simulink model "multiple_generators_els_2018b"  (Simulink 9.2)
settings: Solver=ode15s  StartTime=0.0  StopTime=4000  RelTol=1e-3
InitFcn:
  | global LOData LOModelData gprMdlLP_machine1 gprMdlLP_machine2 gprMdlLP_machine3 gprMdlLP_machine4 gprMdlLP_machine5 significance SteadyState explore explore_signal total_uncertainty
  | load load_opt_multiple_init2.mat
undefined symbols (not defined in the file or in its folder): sigbuilder_block
libraries: simulink x10
settings Model: Creator=Memo Mer  LastModifiedBy=mmercang
settings DataIOCC: LimitDataPoints=off  SaveFormat=Dataset  SignalLoggingSaveFormat=Dataset  ReturnWorkspaceOutputs=on
settings OptimizationCC: LifeSpan=auto
settings DebuggingCC: UnderspecifiedInitializationDetection=Simplified  MergeDetectMultiDrivingBlocksExec=error  FcnCallInpInsideContextMsg=error  StateNameClashWarn=none  SFUnexpectedBacktrackingDiag=error  SFNoUnconditionalDefaultTransitionDiag=error  SFExecutionAtInitializationDiag=warning
settings HardwareCC: ProdBitPerPointer=64  ProdBitPerSizeT=64  ProdBitPerPtrDiffT=64  ProdLargestAtomicFloat=Float  ProdIntDivRoundTo=Zero  ProdEndianess=LittleEndian  ProdWordSize=64  ProdHWDeviceType=Intel->x86-64 (Windows64)
settings ModelReferenceCC: PropagateSignalLabelsOutOfModel=on
settings SFSimCC: SimUseLocalCustomCode=on
settings RTWCC: RTWUseLocalCustomCode=on
settings CodeAppCC: StateflowObjectComments=off
settings GRTTargetCC: TargetLangStandard=C99 (ISO)  CombineOutputUpdateFcns=on  GRTInterface=off
settings ConfigComp: CovMetricSettings=dwe  CovSaveCumulativeToWorkspaceVar=off  CovSaveSingleToWorkspaceVar=off  CovExternalEMLEnable=on

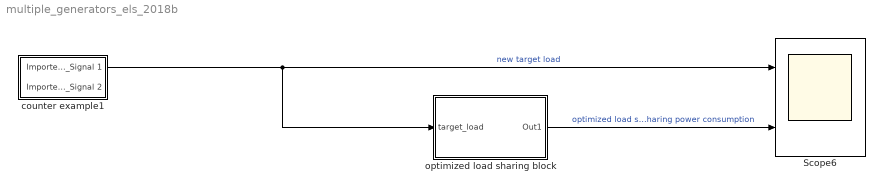
== system multiple_generators_els_2018b ==
  Scope6 : Scope  NumInputPorts=2
  counter example1 : Subsystem  Tag=STV Subsys  LoadFcn=sigbuilder_block('load');  StartFcn=sigbuilder_block('start');  StopFcn=sigbuilder_block('stop');  ClipboardFcn=sigbuilder_block('clipboard');  mask(Sigbuilder block){tuvar=[0:10]}
      mask help: Simulink:masks:SigbuilderBlock_MD
      mask init:
      | if ~strcmp(get_param(bdroot(gcbh),'SimulationStatus'),'stopped') tuvar = sigbuilder_block('maskInit'); end
      settings: CopyFcn=sigbuilder_block('copy');  DeleteFcn=sigbuilder_block('delete');  ModelCloseFcn=sigbuilder_block('modelClose');  PreSaveFcn=sigbuilder_block('preSave');  PauseFcn=sigbuilder_block('pause');  ContinueFcn=sigbuilder_block('continue');  NameChangeFcn=sigbuilder_block('namechange');  OpenFcn=sigbuilder_block('open',[384 46.5 890 699.75 ]);  CloseFcn=sigbuilder_block('close');
      mask Display: plot(0, 0, 100, 100,[2, 2, 32, 32, 2], [68, 8, 8, 68, 68],[32, 2], [38, 38], [32, 19, 2],[53, 60, 44], [32, 17, 17, 2],[16, 16, 31, 31]);txt = getActiveGroup(gcbh);text(2, 100, txt,'verticalAlignment', 'top');
  optimized load sharing block : Subsystem  Tag=equal load sharing
  wires:
  counter example1/1(Imported_Signal 1) -> optimized load sharing block/1(target_load), Scope6/1  "new target load"
  optimized load sharing block/1(Out1) -> Scope6/2  "optimized load sharing power consumption"

== system multiple_generators_els_2018b/counter example1 ==
  Demux : Demux  Tag=STV Demux  Outputs=2
      settings: DisplayOption=none
  FromWs : FromWorkspace  Tag=STV FromWs  VariableName=tuvar  SigBuilderData=DataTag0  VnvData=DataTag1
      SigBuilderData=|
      | common.afterFinalStr = 'Extrapolate'
      | common.sampleTime = '0'
      | dataSet.timeRange = [0 7000]
      | dataSet.name = 'Imported_Group 1'
      | sbobj.Groups.Name = 'Imported_Group 1'
      | sbobj.Groups.Signals(1).Name = 'Imported_Signal 1'
      | sbobj.Groups.Signals(1).XData = [0 1000 1000 2000 2000 3000 4000 4000 5000 5000 6000 6000 7000]
      | sbobj.Groups.Signals(1).YData = [830 830 1035 1035 2500 2500 2500 1830 1830 1170 1170 1660 1660]
      | sbobj.Groups.Signals(2).Name = 'Imported_Signal 2'
      | sbobj.Groups.Signals(2).XData = [0 1000 2000 3000 4000 5000 6000 7000]
      | sbobj.Groups.Signals(2).YData = [1800 1800 1800 1800 1800 1800 1800 1800]
      | sbobj.Groups.TimeRange = [0 7000]
  Imported_Signal 1 : Outport  Tag=STV Outport
  Imported_Signal 2 : Outport  Tag=STV Outport  Port=2
  wires:
  Demux/2 -> Imported_Signal 2/1
  Demux/1 -> Imported_Signal 1/1
  FromWs/1 -> Demux/1

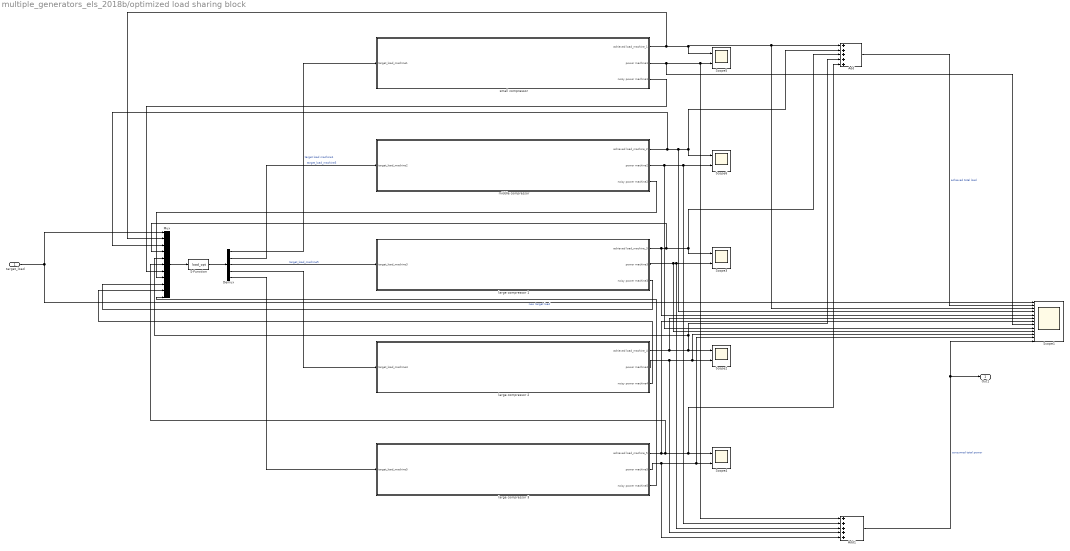
== system multiple_generators_els_2018b/optimized load sharing block ==
  target_load : Inport
  Add : Sum  Inputs=+++++
  Add1 : Sum  Inputs=+++++
  Demux : Demux  Outputs=5
  Mux : Mux  Inputs=11
  S-Function : S-Function  FunctionName=load_opt  Parameters=[],[]  SFunctionDeploymentMode=off  EnableBusSupport=off
  Scope1 : Scope  NumInputPorts=13
  Scope{2..6} (5 alike) : Scope  NumInputPorts=2
  large compressor 1 : Subsystem
  large compressor 2 : Subsystem
  large compressor 3 : Subsystem
  middle compressor : Subsystem
  small compressor : Subsystem
  Out1 : Outport
  wires:
  Add/1 -> Scope1/2  "achieved total load"
  Add1/1 -> Out1/1, Scope1/13  "consumed total power"
  Mux/1 -> S-Function/1
  target_load/1 -> Mux/1, Scope1/1  "new target load"
  S-Function/1 -> Demux/1
  large compressor 1/1(achieved load_machine_3) -> Scope1/5, Mux/4, Scope3/1, Add/3
  large compressor 3/1(achieved load_machine_5) -> Scope1/7, Mux/6, Add/5, Scope4/1
  large compressor 3/2(power machine5) -> Add1/5, Scope1/12, Scope4/2
  middle compressor/1(achieved load_machine_2) -> Scope1/4, Scope6/1, Add/2, Mux/3
  middle compressor/2(power machine2) -> Scope1/9, Add1/2, Scope6/2
  small compressor/2(power machine1) -> Scope1/8, Add1/1, Scope5/2
  Demux/1 -> small compressor/1(target_load_machine1)  "target load machine1"
  Demux/2 -> middle compressor/1(target_load_machine2)  "target_load_machine5"
  Demux/3 -> large compressor 1/1(target_load_machine3)  "target_load_machine5"
  Demux/4 -> large compressor 2/1(target_load_machine4)
  Demux/5 -> large compressor 3/1(target_load_machine5)
  large compressor 3/3(noisy power machine5) -> Mux/11
  large compressor 2/3(noisy power machine4) -> Mux/10
  middle compressor/3(noisy power machine2) -> Mux/8
  large compressor 1/3(noisy power machine3) -> Mux/9
  small compressor/3(noisy power machine1) -> Mux/7
  small compressor/1(achieved load_machine_1) -> Scope5/1, Scope1/3, Add/1, Mux/2
  large compressor 1/2(power machine3) -> Scope1/10, Add1/3, Scope3/2
  large compressor 2/1(achieved load_machine_4) -> Scope1/6, Add/4, Mux/5, Scope2/1
  large compressor 2/2(power machine4) -> Add1/4, Scope1/11, Scope2/2

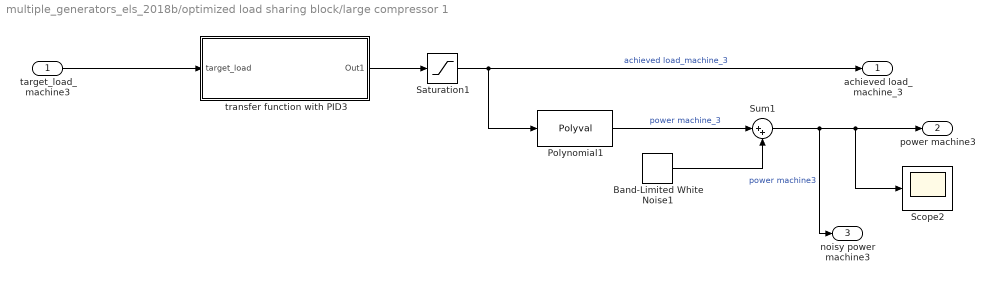
== system multiple_generators_els_2018b/optimized load sharing block/large compressor 1 ==
  target_load_machine3 : Inport
  Band-Limited White Noise1 : simulink/Sources/Band-Limited White Noise  Cov=[0.1]  Ts=5  seed=[23341]
  Polynomial1 : Polyval  Coefs="[-1.53490519e-09  2.28838030e-06 -9.59520873e-04 6.18821903e-01 7.51758182e+01]"
  Saturation1 : Saturate  UpperLimit=795  LowerLimit=194
  Scope2 : Scope
  Sum1 : Sum  Inputs=|++
  transfer function with PID3 : Subsystem
  achieved load_machine_3 : Outport
  power machine3 : Outport  Port=2
  noisy power machine3 : Outport  Port=3
  wires:
  Polynomial1/1 -> Sum1/1  "power machine_3"
  target_load_machine3/1 -> transfer function with PID3/1(target_load)
  transfer function with PID3/1(Out1) -> Saturation1/1
  Band-Limited White Noise1/1 -> Sum1/2
  Saturation1/1 -> achieved load_machine_3/1, Polynomial1/1  "achieved load_machine_3"
  Sum1/1 -> noisy power machine3/1, power machine3/1, Scope2/1  "power machine3"

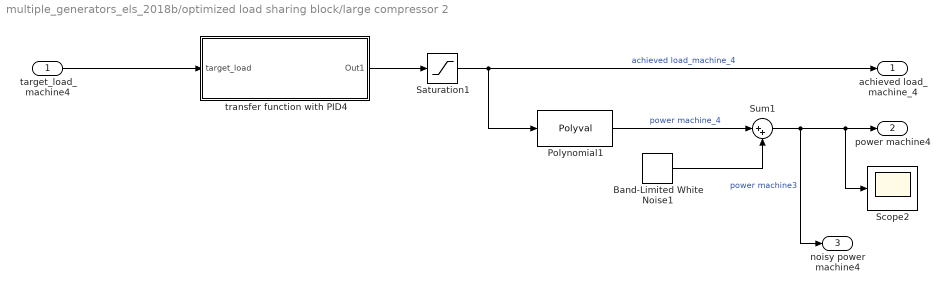
== system multiple_generators_els_2018b/optimized load sharing block/large compressor 2 ==
  target_load_machine4 : Inport
  Band-Limited White Noise1 : simulink/Sources/Band-Limited White Noise  Cov=[0.1]  Ts=5  seed=[23341]
  Polynomial1 : Polyval  Coefs="[-1.53490519e-09  2.28838030e-06 -9.59520873e-04 6.18821903e-01 7.51758182e+01]"
  Saturation1 : Saturate  UpperLimit=795  LowerLimit=194
  Scope2 : Scope
  Sum1 : Sum  Inputs=|++
  transfer function with PID4 : Subsystem
  achieved load_machine_4 : Outport
  power machine4 : Outport  Port=2
  noisy power machine4 : Outport  Port=3
  wires:
  Polynomial1/1 -> Sum1/1  "power machine_4"
  Sum1/1 -> power machine4/1, Scope2/1, noisy power machine4/1  "power machine3"
  target_load_machine4/1 -> transfer function with PID4/1(target_load)
  transfer function with PID4/1(Out1) -> Saturation1/1
  Band-Limited White Noise1/1 -> Sum1/2
  Saturation1/1 -> achieved load_machine_4/1, Polynomial1/1  "achieved load_machine_4"

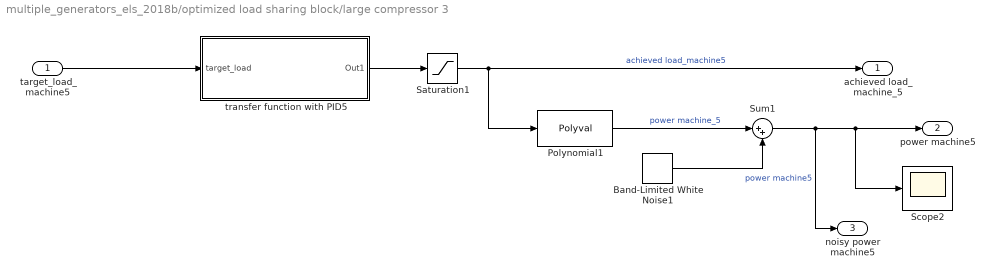
== system multiple_generators_els_2018b/optimized load sharing block/large compressor 3 ==
  target_load_machine5 : Inport
  Band-Limited White Noise1 : simulink/Sources/Band-Limited White Noise  Cov=[0.1]  Ts=5  seed=[23341]
  Polynomial1 : Polyval  Coefs="[-1.53490519e-09  2.28838030e-06 -9.59520873e-04 6.18821903e-01 7.51758182e+01]"
  Saturation1 : Saturate  UpperLimit=795  LowerLimit=194
  Scope2 : Scope
  Sum1 : Sum  Inputs=|++
  transfer function with PID5 : Subsystem
  achieved load_machine_5 : Outport
  power machine5 : Outport  Port=2
  noisy power machine5 : Outport  Port=3
  wires:
  Polynomial1/1 -> Sum1/1  "power machine_5"
  target_load_machine5/1 -> transfer function with PID5/1(target_load)
  transfer function with PID5/1(Out1) -> Saturation1/1
  Band-Limited White Noise1/1 -> Sum1/2
  Saturation1/1 -> achieved load_machine_5/1, Polynomial1/1  "achieved load_machine5"
  Sum1/1 -> power machine5/1, Scope2/1, noisy power machine5/1  "power machine5"

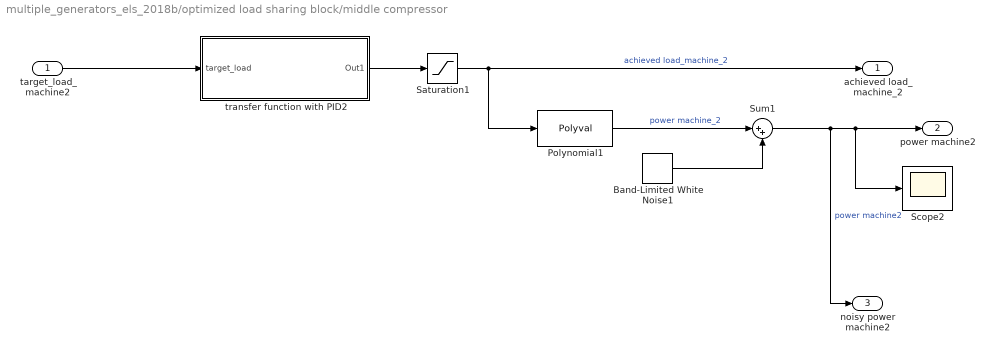
== system multiple_generators_els_2018b/optimized load sharing block/middle compressor ==
  target_load_machine2 : Inport
  Band-Limited White Noise1 : simulink/Sources/Band-Limited White Noise  Cov=[0.1]  Ts=5  seed=[23341]
  Polynomial1 : Polyval  Coefs=[-1.42718017e-08 1.87477980e-05 -8.28649653e-03 1.88469092 -2.19952823]
  Saturation1 : Saturate  UpperLimit=537  LowerLimit=237
  Scope2 : Scope
  Sum1 : Sum  Inputs=|++
  transfer function with PID2 : Subsystem
  achieved load_machine_2 : Outport
  power machine2 : Outport  Port=2
  noisy power machine2 : Outport  Port=3
  wires:
  Polynomial1/1 -> Sum1/1  "power machine_2"
  target_load_machine2/1 -> transfer function with PID2/1(target_load)
  transfer function with PID2/1(Out1) -> Saturation1/1
  Band-Limited White Noise1/1 -> Sum1/2
  Saturation1/1 -> achieved load_machine_2/1, Polynomial1/1  "achieved load_machine_2"
  Sum1/1 -> noisy power machine2/1, power machine2/1, Scope2/1  "power machine2"

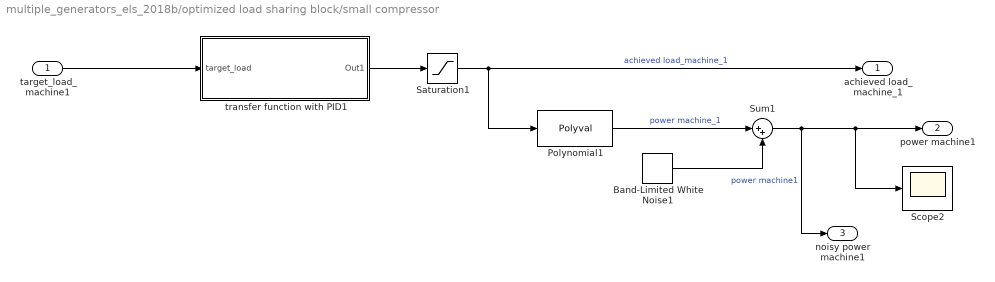
== system multiple_generators_els_2018b/optimized load sharing block/small compressor ==
  target_load_machine1 : Inport
  Band-Limited White Noise1 : simulink/Sources/Band-Limited White Noise  Cov=[0.1]  Ts=5  seed=[23341]
  Polynomial1 : Polyval  Coefs=[-9e-08 4e-05 -0.0052 0.7765 15.661]
  Saturation1 : Saturate  UpperLimit=220  LowerLimit=56
  Scope2 : Scope
  Sum1 : Sum  Inputs=|++
  transfer function with PID1 : Subsystem
  achieved load_machine_1 : Outport
  power machine1 : Outport  Port=2
  noisy power machine1 : Outport  Port=3
  wires:
  Polynomial1/1 -> Sum1/1  "power machine_1"
  target_load_machine1/1 -> transfer function with PID1/1(target_load)
  transfer function with PID1/1(Out1) -> Saturation1/1
  Band-Limited White Noise1/1 -> Sum1/2
  Saturation1/1 -> achieved load_machine_1/1, Polynomial1/1  "achieved load_machine_1"
  Sum1/1 -> power machine1/1, Scope2/1, noisy power machine1/1  "power machine1"

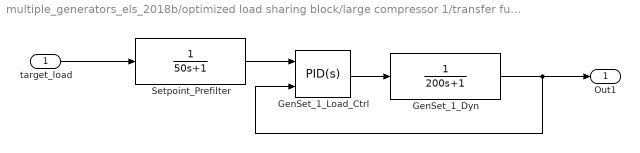
== system multiple_generators_els_2018b/optimized load sharing block/large compressor 1/transfer function with PID3 ==
  target_load : Inport
  GenSet_1_Dyn : TransferFcn  Denominator=[200 1]
  GenSet_1_Load_Ctrl : simulink/Continuous/PID Controller (2DOF)  Controller=PID  Form=Parallel  TimeDomain=Continuous-time  SampleTime=-1  IntegratorMethod=Forward Euler  FilterMethod=Forward Euler  ControllerParametersSource=internal  P=100  I=10  D=0  UseFilter=on  N=100  b=1  c=1  TunerSelectOption=Transfer Function Based (PID Tuner App)  InitialConditionSource=internal  InitialConditionForIntegrator=0  InitialConditionForFilter=0  DifferentiatorICPrevScaledInput=0  ExternalReset=none  TrackingMode=off  Kt=1  LimitOutput=off  UpperSaturationLimit=inf  LowerSaturationLimit=-inf  LinearizeAsGain=on  AntiWindupMode=none  Kb=1  POutMin=[]  POutMax=[]  IOutMin=[]  IOutMax=[]  DOutMin=[]  DOutMax=[]  NOutMin=[]  NOutMax=[]  bOutMin=[]  bOutMax=[]  cOutMin=[]  cOutMax=[]  SumOutMin=[]  SumOutMax=[]  SaturationOutMin=[]  SaturationOutMax=[]  PParamMin=[]  PParamMax=[]  IParamMin=[]  IParamMax=[]  DParamMin=[]  DParamMax=[]  NParamMin=[]  NParamMax=[]  bParamMin=[]  bParamMax=[]  cParamMin=[]  cParamMax=[]  KbParamMin=[]  KbParamMax=[]  KtParamMin=[]  KtParamMax=[]  KbOutMin=[]  KbOutMax=[]  KtOutMin=[]  KtOutMax=[]  IntegratorOutMin=[]  IntegratorOutMax=[]  FilterOutMin=[]  FilterOutMax=[]  SumI1OutMin=[]  SumI1OutMax=[]  SumI2OutMin=[]  SumI2OutMax=[]  SumI3OutMin=[]  SumI3OutMax=[]  SumI4OutMin=[]  SumI4OutMax=[]  SumDOutMin=[]  SumDOutMax=[]  Sum1OutMin=[]  Sum1OutMax=[]  Sum2OutMin=[]  Sum2OutMax=[]  Sum3OutMin=[]  Sum3OutMax=[]  DifferentiatorOutMin=[]  DifferentiatorOutMax=[]  FilterDiffOutCoefMin=[]  FilterDiffOutCoefMax=[]  ReciprocalOutMin=[]  ReciprocalOutMax=[]  SumDenOutMin=[]  SumDenOutMax=[]  SumNumOutMin=[]  SumNumOutMax=[]  DivideOutMin=[]  DivideOutMax=[]  IntegratorContinuousStateAttributes=''  IntegratorStateMustResolveToSignalObject=off  IntegratorRTWStateStorageClass=Auto  FilterContinuousStateAttributes=''  FilterStateMustResolveToSignalObject=off  FilterRTWStateStorageClass=Auto  ParallelPVariant=InternalParameters  IdealPVariant=Disabled  IVariant=InternalParameters  DVariant=InternalParameters  bVariant=InternalParameters  cVariant=InternalParameters  IntegratorVariant=Continuous  SatVariant=Disabled  AWVariant=Passthrough  PCopyVariant=Disabled  TRVariant=Disabled  FdbkBlocksVariant=Forward  IdealPFdbkVariant=Disabled  SatFdbkVariant=Disabled  DerivativeFilterVariant=ContFilter  NVariant=InternalParameters  NCopyVariant=Disabled  FilterICVariant=InternalICsFilter  IntegratorICVariant=InternalICs  ExternalResetVariant=Disabled  TRSumVariant=Passthrough  SumFdbkVariant=Disabled  SumVariant=Sum_PID
  Setpoint_Prefilter : TransferFcn  Denominator=[50 1]
  Out1 : Outport
  wires:
  GenSet_1_Load_Ctrl/1 -> GenSet_1_Dyn/1
  Setpoint_Prefilter/1 -> GenSet_1_Load_Ctrl/1
  target_load/1 -> Setpoint_Prefilter/1
  GenSet_1_Dyn/1 -> Out1/1, GenSet_1_Load_Ctrl/2

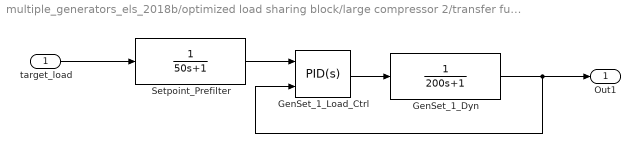
== system multiple_generators_els_2018b/optimized load sharing block/large compressor 2/transfer function with PID4 ==
  target_load : Inport
  GenSet_1_Dyn : TransferFcn  Denominator=[200 1]
  GenSet_1_Load_Ctrl : simulink/Continuous/PID Controller (2DOF)  Controller=PID  Form=Parallel  TimeDomain=Continuous-time  SampleTime=-1  IntegratorMethod=Forward Euler  FilterMethod=Forward Euler  ControllerParametersSource=internal  P=100  I=10  D=0  UseFilter=on  N=100  b=1  c=1  TunerSelectOption=Transfer Function Based (PID Tuner App)  InitialConditionSource=internal  InitialConditionForIntegrator=0  InitialConditionForFilter=0  DifferentiatorICPrevScaledInput=0  ExternalReset=none  TrackingMode=off  Kt=1  LimitOutput=off  UpperSaturationLimit=inf  LowerSaturationLimit=-inf  LinearizeAsGain=on  AntiWindupMode=none  Kb=1  POutMin=[]  POutMax=[]  IOutMin=[]  IOutMax=[]  DOutMin=[]  DOutMax=[]  NOutMin=[]  NOutMax=[]  bOutMin=[]  bOutMax=[]  cOutMin=[]  cOutMax=[]  SumOutMin=[]  SumOutMax=[]  SaturationOutMin=[]  SaturationOutMax=[]  PParamMin=[]  PParamMax=[]  IParamMin=[]  IParamMax=[]  DParamMin=[]  DParamMax=[]  NParamMin=[]  NParamMax=[]  bParamMin=[]  bParamMax=[]  cParamMin=[]  cParamMax=[]  KbParamMin=[]  KbParamMax=[]  KtParamMin=[]  KtParamMax=[]  KbOutMin=[]  KbOutMax=[]  KtOutMin=[]  KtOutMax=[]  IntegratorOutMin=[]  IntegratorOutMax=[]  FilterOutMin=[]  FilterOutMax=[]  SumI1OutMin=[]  SumI1OutMax=[]  SumI2OutMin=[]  SumI2OutMax=[]  SumI3OutMin=[]  SumI3OutMax=[]  SumI4OutMin=[]  SumI4OutMax=[]  SumDOutMin=[]  SumDOutMax=[]  Sum1OutMin=[]  Sum1OutMax=[]  Sum2OutMin=[]  Sum2OutMax=[]  Sum3OutMin=[]  Sum3OutMax=[]  DifferentiatorOutMin=[]  DifferentiatorOutMax=[]  FilterDiffOutCoefMin=[]  FilterDiffOutCoefMax=[]  ReciprocalOutMin=[]  ReciprocalOutMax=[]  SumDenOutMin=[]  SumDenOutMax=[]  SumNumOutMin=[]  SumNumOutMax=[]  DivideOutMin=[]  DivideOutMax=[]  IntegratorContinuousStateAttributes=''  IntegratorStateMustResolveToSignalObject=off  IntegratorRTWStateStorageClass=Auto  FilterContinuousStateAttributes=''  FilterStateMustResolveToSignalObject=off  FilterRTWStateStorageClass=Auto  ParallelPVariant=InternalParameters  IdealPVariant=Disabled  IVariant=InternalParameters  DVariant=InternalParameters  bVariant=InternalParameters  cVariant=InternalParameters  IntegratorVariant=Continuous  SatVariant=Disabled  AWVariant=Passthrough  PCopyVariant=Disabled  TRVariant=Disabled  FdbkBlocksVariant=Forward  IdealPFdbkVariant=Disabled  SatFdbkVariant=Disabled  DerivativeFilterVariant=ContFilter  NVariant=InternalParameters  NCopyVariant=Disabled  FilterICVariant=InternalICsFilter  IntegratorICVariant=InternalICs  ExternalResetVariant=Disabled  TRSumVariant=Passthrough  SumFdbkVariant=Disabled  SumVariant=Sum_PID
  Setpoint_Prefilter : TransferFcn  Denominator=[50 1]
  Out1 : Outport
  wires:
  GenSet_1_Load_Ctrl/1 -> GenSet_1_Dyn/1
  Setpoint_Prefilter/1 -> GenSet_1_Load_Ctrl/1
  target_load/1 -> Setpoint_Prefilter/1
  GenSet_1_Dyn/1 -> Out1/1, GenSet_1_Load_Ctrl/2

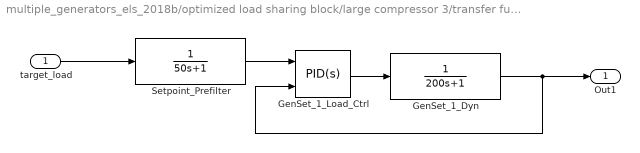
== system multiple_generators_els_2018b/optimized load sharing block/large compressor 3/transfer function with PID5 ==
  target_load : Inport
  GenSet_1_Dyn : TransferFcn  Denominator=[200 1]
  GenSet_1_Load_Ctrl : simulink/Continuous/PID Controller (2DOF)  Controller=PID  Form=Parallel  TimeDomain=Continuous-time  SampleTime=-1  IntegratorMethod=Forward Euler  FilterMethod=Forward Euler  ControllerParametersSource=internal  P=100  I=10  D=0  UseFilter=on  N=100  b=1  c=1  TunerSelectOption=Transfer Function Based (PID Tuner App)  InitialConditionSource=internal  InitialConditionForIntegrator=0  InitialConditionForFilter=0  DifferentiatorICPrevScaledInput=0  ExternalReset=none  TrackingMode=off  Kt=1  LimitOutput=off  UpperSaturationLimit=inf  LowerSaturationLimit=-inf  LinearizeAsGain=on  AntiWindupMode=none  Kb=1  POutMin=[]  POutMax=[]  IOutMin=[]  IOutMax=[]  DOutMin=[]  DOutMax=[]  NOutMin=[]  NOutMax=[]  bOutMin=[]  bOutMax=[]  cOutMin=[]  cOutMax=[]  SumOutMin=[]  SumOutMax=[]  SaturationOutMin=[]  SaturationOutMax=[]  PParamMin=[]  PParamMax=[]  IParamMin=[]  IParamMax=[]  DParamMin=[]  DParamMax=[]  NParamMin=[]  NParamMax=[]  bParamMin=[]  bParamMax=[]  cParamMin=[]  cParamMax=[]  KbParamMin=[]  KbParamMax=[]  KtParamMin=[]  KtParamMax=[]  KbOutMin=[]  KbOutMax=[]  KtOutMin=[]  KtOutMax=[]  IntegratorOutMin=[]  IntegratorOutMax=[]  FilterOutMin=[]  FilterOutMax=[]  SumI1OutMin=[]  SumI1OutMax=[]  SumI2OutMin=[]  SumI2OutMax=[]  SumI3OutMin=[]  SumI3OutMax=[]  SumI4OutMin=[]  SumI4OutMax=[]  SumDOutMin=[]  SumDOutMax=[]  Sum1OutMin=[]  Sum1OutMax=[]  Sum2OutMin=[]  Sum2OutMax=[]  Sum3OutMin=[]  Sum3OutMax=[]  DifferentiatorOutMin=[]  DifferentiatorOutMax=[]  FilterDiffOutCoefMin=[]  FilterDiffOutCoefMax=[]  ReciprocalOutMin=[]  ReciprocalOutMax=[]  SumDenOutMin=[]  SumDenOutMax=[]  SumNumOutMin=[]  SumNumOutMax=[]  DivideOutMin=[]  DivideOutMax=[]  IntegratorContinuousStateAttributes=''  IntegratorStateMustResolveToSignalObject=off  IntegratorRTWStateStorageClass=Auto  FilterContinuousStateAttributes=''  FilterStateMustResolveToSignalObject=off  FilterRTWStateStorageClass=Auto  ParallelPVariant=InternalParameters  IdealPVariant=Disabled  IVariant=InternalParameters  DVariant=InternalParameters  bVariant=InternalParameters  cVariant=InternalParameters  IntegratorVariant=Continuous  SatVariant=Disabled  AWVariant=Passthrough  PCopyVariant=Disabled  TRVariant=Disabled  FdbkBlocksVariant=Forward  IdealPFdbkVariant=Disabled  SatFdbkVariant=Disabled  DerivativeFilterVariant=ContFilter  NVariant=InternalParameters  NCopyVariant=Disabled  FilterICVariant=InternalICsFilter  IntegratorICVariant=InternalICs  ExternalResetVariant=Disabled  TRSumVariant=Passthrough  SumFdbkVariant=Disabled  SumVariant=Sum_PID
  Setpoint_Prefilter : TransferFcn  Denominator=[50 1]
  Out1 : Outport
  wires:
  GenSet_1_Load_Ctrl/1 -> GenSet_1_Dyn/1
  Setpoint_Prefilter/1 -> GenSet_1_Load_Ctrl/1
  target_load/1 -> Setpoint_Prefilter/1
  GenSet_1_Dyn/1 -> Out1/1, GenSet_1_Load_Ctrl/2

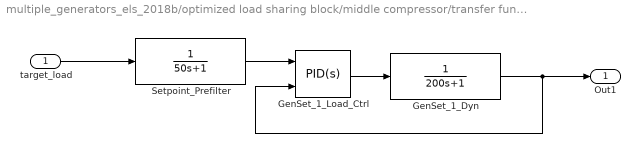
== system multiple_generators_els_2018b/optimized load sharing block/middle compressor/transfer function with PID2 ==
  target_load : Inport
  GenSet_1_Dyn : TransferFcn  Denominator=[200 1]
  GenSet_1_Load_Ctrl : simulink/Continuous/PID Controller (2DOF)  Controller=PID  Form=Parallel  TimeDomain=Continuous-time  SampleTime=-1  IntegratorMethod=Forward Euler  FilterMethod=Forward Euler  ControllerParametersSource=internal  P=100  I=10  D=0  UseFilter=on  N=100  b=1  c=1  TunerSelectOption=Transfer Function Based (PID Tuner App)  InitialConditionSource=internal  InitialConditionForIntegrator=0  InitialConditionForFilter=0  DifferentiatorICPrevScaledInput=0  ExternalReset=none  TrackingMode=off  Kt=1  LimitOutput=off  UpperSaturationLimit=inf  LowerSaturationLimit=-inf  LinearizeAsGain=on  AntiWindupMode=none  Kb=1  POutMin=[]  POutMax=[]  IOutMin=[]  IOutMax=[]  DOutMin=[]  DOutMax=[]  NOutMin=[]  NOutMax=[]  bOutMin=[]  bOutMax=[]  cOutMin=[]  cOutMax=[]  SumOutMin=[]  SumOutMax=[]  SaturationOutMin=[]  SaturationOutMax=[]  PParamMin=[]  PParamMax=[]  IParamMin=[]  IParamMax=[]  DParamMin=[]  DParamMax=[]  NParamMin=[]  NParamMax=[]  bParamMin=[]  bParamMax=[]  cParamMin=[]  cParamMax=[]  KbParamMin=[]  KbParamMax=[]  KtParamMin=[]  KtParamMax=[]  KbOutMin=[]  KbOutMax=[]  KtOutMin=[]  KtOutMax=[]  IntegratorOutMin=[]  IntegratorOutMax=[]  FilterOutMin=[]  FilterOutMax=[]  SumI1OutMin=[]  SumI1OutMax=[]  SumI2OutMin=[]  SumI2OutMax=[]  SumI3OutMin=[]  SumI3OutMax=[]  SumI4OutMin=[]  SumI4OutMax=[]  SumDOutMin=[]  SumDOutMax=[]  Sum1OutMin=[]  Sum1OutMax=[]  Sum2OutMin=[]  Sum2OutMax=[]  Sum3OutMin=[]  Sum3OutMax=[]  DifferentiatorOutMin=[]  DifferentiatorOutMax=[]  FilterDiffOutCoefMin=[]  FilterDiffOutCoefMax=[]  ReciprocalOutMin=[]  ReciprocalOutMax=[]  SumDenOutMin=[]  SumDenOutMax=[]  SumNumOutMin=[]  SumNumOutMax=[]  DivideOutMin=[]  DivideOutMax=[]  IntegratorContinuousStateAttributes=''  IntegratorStateMustResolveToSignalObject=off  IntegratorRTWStateStorageClass=Auto  FilterContinuousStateAttributes=''  FilterStateMustResolveToSignalObject=off  FilterRTWStateStorageClass=Auto  ParallelPVariant=InternalParameters  IdealPVariant=Disabled  IVariant=InternalParameters  DVariant=InternalParameters  bVariant=InternalParameters  cVariant=InternalParameters  IntegratorVariant=Continuous  SatVariant=Disabled  AWVariant=Passthrough  PCopyVariant=Disabled  TRVariant=Disabled  FdbkBlocksVariant=Forward  IdealPFdbkVariant=Disabled  SatFdbkVariant=Disabled  DerivativeFilterVariant=ContFilter  NVariant=InternalParameters  NCopyVariant=Disabled  FilterICVariant=InternalICsFilter  IntegratorICVariant=InternalICs  ExternalResetVariant=Disabled  TRSumVariant=Passthrough  SumFdbkVariant=Disabled  SumVariant=Sum_PID
  Setpoint_Prefilter : TransferFcn  Denominator=[50 1]
  Out1 : Outport
  wires:
  GenSet_1_Load_Ctrl/1 -> GenSet_1_Dyn/1
  Setpoint_Prefilter/1 -> GenSet_1_Load_Ctrl/1
  target_load/1 -> Setpoint_Prefilter/1
  GenSet_1_Dyn/1 -> Out1/1, GenSet_1_Load_Ctrl/2

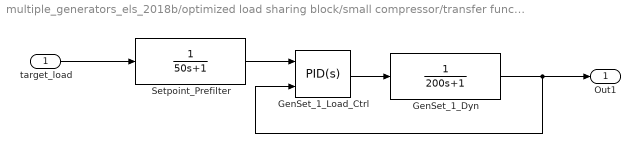
== system multiple_generators_els_2018b/optimized load sharing block/small compressor/transfer function with PID1 ==
  target_load : Inport
  GenSet_1_Dyn : TransferFcn  Denominator=[200 1]
  GenSet_1_Load_Ctrl : simulink/Continuous/PID Controller (2DOF)  Controller=PID  Form=Parallel  TimeDomain=Continuous-time  SampleTime=-1  IntegratorMethod=Forward Euler  FilterMethod=Forward Euler  ControllerParametersSource=internal  P=100  I=10  D=0  UseFilter=on  N=100  b=1  c=1  TunerSelectOption=Transfer Function Based (PID Tuner App)  InitialConditionSource=internal  InitialConditionForIntegrator=0  InitialConditionForFilter=0  DifferentiatorICPrevScaledInput=0  ExternalReset=none  TrackingMode=off  Kt=1  LimitOutput=off  UpperSaturationLimit=inf  LowerSaturationLimit=-inf  LinearizeAsGain=on  AntiWindupMode=none  Kb=1  POutMin=[]  POutMax=[]  IOutMin=[]  IOutMax=[]  DOutMin=[]  DOutMax=[]  NOutMin=[]  NOutMax=[]  bOutMin=[]  bOutMax=[]  cOutMin=[]  cOutMax=[]  SumOutMin=[]  SumOutMax=[]  SaturationOutMin=[]  SaturationOutMax=[]  PParamMin=[]  PParamMax=[]  IParamMin=[]  IParamMax=[]  DParamMin=[]  DParamMax=[]  NParamMin=[]  NParamMax=[]  bParamMin=[]  bParamMax=[]  cParamMin=[]  cParamMax=[]  KbParamMin=[]  KbParamMax=[]  KtParamMin=[]  KtParamMax=[]  KbOutMin=[]  KbOutMax=[]  KtOutMin=[]  KtOutMax=[]  IntegratorOutMin=[]  IntegratorOutMax=[]  FilterOutMin=[]  FilterOutMax=[]  SumI1OutMin=[]  SumI1OutMax=[]  SumI2OutMin=[]  SumI2OutMax=[]  SumI3OutMin=[]  SumI3OutMax=[]  SumI4OutMin=[]  SumI4OutMax=[]  SumDOutMin=[]  SumDOutMax=[]  Sum1OutMin=[]  Sum1OutMax=[]  Sum2OutMin=[]  Sum2OutMax=[]  Sum3OutMin=[]  Sum3OutMax=[]  DifferentiatorOutMin=[]  DifferentiatorOutMax=[]  FilterDiffOutCoefMin=[]  FilterDiffOutCoefMax=[]  ReciprocalOutMin=[]  ReciprocalOutMax=[]  SumDenOutMin=[]  SumDenOutMax=[]  SumNumOutMin=[]  SumNumOutMax=[]  DivideOutMin=[]  DivideOutMax=[]  IntegratorContinuousStateAttributes=''  IntegratorStateMustResolveToSignalObject=off  IntegratorRTWStateStorageClass=Auto  FilterContinuousStateAttributes=''  FilterStateMustResolveToSignalObject=off  FilterRTWStateStorageClass=Auto  ParallelPVariant=InternalParameters  IdealPVariant=Disabled  IVariant=InternalParameters  DVariant=InternalParameters  bVariant=InternalParameters  cVariant=InternalParameters  IntegratorVariant=Continuous  SatVariant=Disabled  AWVariant=Passthrough  PCopyVariant=Disabled  TRVariant=Disabled  FdbkBlocksVariant=Forward  IdealPFdbkVariant=Disabled  SatFdbkVariant=Disabled  DerivativeFilterVariant=ContFilter  NVariant=InternalParameters  NCopyVariant=Disabled  FilterICVariant=InternalICsFilter  IntegratorICVariant=InternalICs  ExternalResetVariant=Disabled  TRSumVariant=Passthrough  SumFdbkVariant=Disabled  SumVariant=Sum_PID
  Setpoint_Prefilter : TransferFcn  Denominator=[50 1]
  Out1 : Outport
  wires:
  GenSet_1_Load_Ctrl/1 -> GenSet_1_Dyn/1
  Setpoint_Prefilter/1 -> GenSet_1_Load_Ctrl/1
  target_load/1 -> Setpoint_Prefilter/1
  GenSet_1_Dyn/1 -> Out1/1, GenSet_1_Load_Ctrl/2
